simulink library "RGP_ctrl"  (R2020a)
settings: Solver=VariableStepAuto  StartTime=0.0  StopTime=10.0  RelTol=1e-3
undefined symbols (not defined in the file or in its folder): postVarGain, predMeanGain, xBasis
libraries: dspsigops x2, calcUCB x1
settings Model: Creator=Ayaz  LastModifiedBy=Ayaz

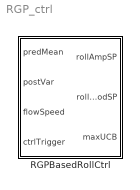
== system RGP_ctrl ==
  RGPBasedRollCtrl : Subsystem  mask{predMeanGain=predMeanGain, postVarGain=postVarGain, xBasis=xBasis, initRollAmpDeg=0, initRollPeriodSec=20}
      mask prompts: predMeanGain "Prediction mean gain"; postVarGain "Posterior variance gain"; xBasis "Basis vector"; initRollAmpDeg "Initial roll amplitude [deg]"; initRollPeriodSec "Initial roll period [sec]"
      mask TypeOptions predMeanGain: Subsystem/predMeanGain
      mask TypeOptions postVarGain: Subsystem/postVarGain
      mask TypeOptions xBasis: Subsystem/xBasis
      mask TypeOptions initRollAmpDeg:
      | Sample
      | and Hold/initCond
      mask TypeOptions initRollPeriodSec:
      | Sample
      | and Hold1/initCond

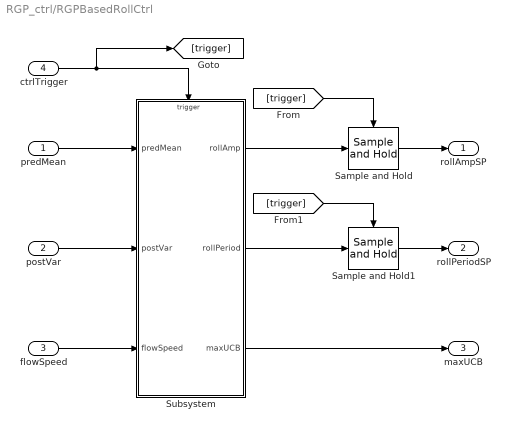
== system RGP_ctrl/RGPBasedRollCtrl ==
  predMean : Inport
  postVar : Inport  Port=2
  flowSpeed : Inport  Port=3
  ctrlTrigger : Inport  Port=4
  Sample and Hold : dspsigops/Sample and Hold  trig=Rising edge  initCond=initRollAmpDeg  latchinput=off
  Sample and Hold1 : dspsigops/Sample and Hold  trig=Rising edge  initCond=initRollPeriodSec  latchinput=off
  Subsystem : Subsystem  mask{predMeanGain=predMeanGain, postVarGain=postVarGain, xBasis=xBasis}
      mask prompts: predMeanGain "Prediction mean gain"; postVarGain "Posterior variance gain"; xBasis "Basis vector"
      mask TypeOptions predMeanGain: UCB/predMeanGain
      mask TypeOptions postVarGain: UCB/postVarGain
      mask TypeOptions xBasis: Constant/Value
  rollAmpSP : Outport
  rollPeriodSP : Outport  Port=2
  maxUCB : Outport  Port=3
  wires:
  predMean/1 -> Subsystem/1(predMean)
  postVar/1 -> Subsystem/2(postVar)
  flowSpeed/1 -> Subsystem/3(flowSpeed)
  Subsystem/2(rollPeriod) -> Sample and Hold1/1
  Sample and Hold/1 -> rollAmpSP/1
  Subsystem/3(maxUCB) -> maxUCB/1
  Subsystem/1(rollAmp) -> Sample and Hold/1
  Sample and Hold1/1 -> rollPeriodSP/1
  ctrlTrigger/1 -> [trigger], Subsystem/Trigger
  [trigger] -> Sample and Hold/Trigger
  [trigger] -> Sample and Hold1/Trigger

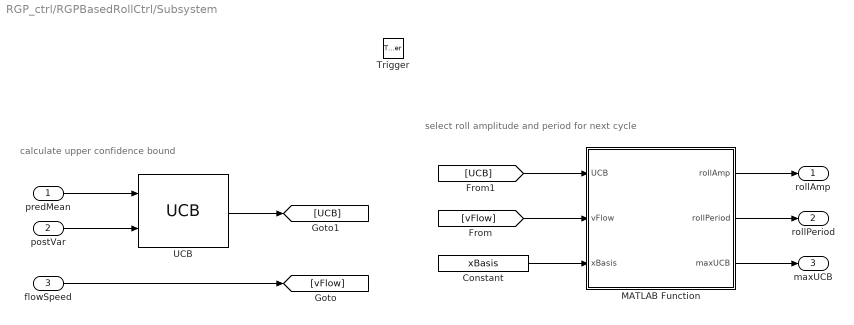
== system RGP_ctrl/RGPBasedRollCtrl/Subsystem ==
  note: select roll amplitude and period for next cycle
  note: calculate upper confidence bound
  predMean : Inport
  postVar : Inport  Port=2
  flowSpeed : Inport  Port=3
  Trigger : TriggerPort  VariantControl=Variant
  Constant : Constant  Value=xBasis  VectorParams1D=off
  MATLAB Function : MATLAB Function  TreatAsAtomicUnit=on
  UCB : calcUCB/UCB  predMeanGain=predMeanGain  postVarGain=postVarGain
  rollAmp : Outport
  rollPeriod : Outport  Port=2
  maxUCB : Outport  Port=3
  wires:
  predMean/1 -> UCB/1
  postVar/1 -> UCB/2
  flowSpeed/1 -> [vFlow]
  UCB/1 -> [UCB]
  [UCB] -> MATLAB Function/1(UCB)
  [vFlow] -> MATLAB Function/2(vFlow)
  Constant/1 -> MATLAB Function/3(xBasis)
  MATLAB Function/1(rollAmp) -> rollAmp/1
  MATLAB Function/2(rollPeriod) -> rollPeriod/1
  MATLAB Function/3(maxUCB) -> maxUCB/1

== matlab function RGP_ctrl/RGPBasedRollCtrl/Subsystem/MATLAB Function ==
  data: UCB input; rollAmp output; vFlow input; xBasis input; rollPeriod output; maxUCB output
function [rollAmp,rollPeriod,maxUCB] = ...
    selectRollAmpAndPeriod(UCB,vFlow,xBasis)

[rollAmp,rollPeriod,maxUCB] = selectRollAmpAndPeriod(UCB,vFlow,xBasis);

end
